simulink model "ROPOD_Control_Control_SIM"  (R2017b)
settings: Solver=VariableStepAuto  StartTime=0.0  StopTime=inf  RelTol=1e-3
values from neighbouring files (symbols this model uses):
  FFtheta_intia = 0    [init_model.m]
  FFxy_mass = 0*80    (= 0)    [init_model.m]
  flock_FFtheta_friction = 50    [init_model.m]
  flock_FFxy_friction = 100    [init_model.m]
  I_fhz_ddelta_cntr = 0    [init_model.m]
  I_fhz_dtheta_cntr = 0.3    [init_model.m]
  I_fhz_dtheta_flock_cntr = 0.1    [init_model.m]
  I_fhz_dvarphi_cntr = 0    [init_model.m]
  I_fhz_dxdy_cntr = 0.25    [init_model.m]
  I_fhz_dxdy_flock_cntr = 0.1    [init_model.m]
  K_gain_ddelta_cntr = 0.1    [init_model.m]
  K_gain_dtheta_cntr = 150    [init_model.m]
  K_gain_dtheta_flock_cntr = 100    [init_model.m]
  K_gain_dvarphi_cntr = 0.05    [init_model.m]
  K_gain_dxdy_cntr = 200    [init_model.m]
  K_gain_dxdy_flock_cntr = 200    [init_model.m]
  LL_wp_fhz_ddelta_cntr = 2    [init_model.m]
  LL_wp_fhz_dtheta_cntr = 20    [init_model.m]
  LL_wp_fhz_dtheta_flock_cntr = 20    [init_model.m]
  LL_wp_fhz_dvarphi_cntr = 10    [init_model.m]
  LL_wp_fhz_dxdy_cntr = 20    [init_model.m]
  LL_wp_fhz_dxdy_flock_cntr = 20    [init_model.m]
  LL_wz_fhz_ddelta_cntr = 2    [init_model.m]
  LL_wz_fhz_dtheta_cntr = 20    [init_model.m]
  LL_wz_fhz_dtheta_flock_cntr = 20    [init_model.m]
  LL_wz_fhz_dvarphi_cntr = 2    [init_model.m]
  LL_wz_fhz_dxdy_cntr = 20    [init_model.m]
  LL_wz_fhz_dxdy_flock_cntr = 20    [init_model.m]
  LPF_fhz_ddelta_cntr = 50    [init_model.m]
  LPF_fhz_ddelta_meas = 50    [init_model.m]
  LPF_fhz_dtheta_cntr = 100    [init_model.m]
  LPF_fhz_dtheta_flock_cntr = 40    [init_model.m]
  LPF_fhz_dvarphi_cntr = 50    [init_model.m]
  LPF_fhz_dvarphi_meas = 50    [init_model.m]
  LPF_fhz_dxdy_cntr = 100    [init_model.m]
  LPF_fhz_dxdy_flock_cntr = 40    [init_model.m]
  max_flock_acc_theta = 0.5    [init_model.m]
  max_flock_acc_xy = 0.5    [init_model.m]
  max_flock_vel_theta = 1.0    (= 1)    [init_model.m]
  max_flock_vel_xy = 1.0    (= 1)    [init_model.m]
  max_hw_tau = 7.0    (= 7)    [init_model.m]
  max_ropod_acc_theta = 1.6    [init_model.m]
  max_ropod_acc_xy = 2.0    (= 2)    [init_model.m]
  max_ropod_sw_force = 500    [init_model.m]
  max_ropod_sw_tau = 250    [init_model.m]
  max_ropod_vel_theta = 1.6    [init_model.m]
  max_ropod_vel_xy = 2.0    (= 2)    [init_model.m]
  max_sw_current = 10    [init_model.m]
  Nagents = 2    [init_model.m]
  Nwheels = 4    [Jqwl_numeric_function.m]    (also in S_matrix.m; extract_kinmodel_parameters.m; init_model.m; tau_optimal_dist_vec_fun.m)
  pivot_offs_sws = [0.0243    0.4689    0.3384    5.9050]    [init_model.m]
  ropod_kinmodel_pv = struct2array(ropod_kinmodel_param)    [set_ropod_KinModparams.m]
  ropod_position_inflock = [-1 0 3.1416]    [init_model.m]
  SW_COM1_ENABLE1 = hex2dec('0001')    [init_model.m]
  SW_COM1_ENABLE2 = hex2dec('0002')    [init_model.m]
  SW_COM1_MODE_TORQUE = bitshift(hex2dec('0000'),2)    [init_model.m]
  SW_COM1_MODE_VELOCITY = bitshift(hex2dec('0002'),2)    [init_model.m]
  SW_COM1_USE_TS = hex2dec('8000')    [init_model.m]
  Tinit = 2    [init_model.m]
  Ts = 0.001    [init_model.m]
  Tsflck = 0.01    [init_model.m]
undefined symbols (not defined in the file or in its folder): DiscIntNeverNeededParam, sw_tau_2_curr
libraries: simulink x80, cstblocks x30, dspsigops x12, dspnetwork x4
(part 1 of 6)
settings Model: Creator=cesar  LastModifiedBy=cesar
settings OptimizationCC: DefaultParameterBehavior=Inlined  UseFloatMulNetSlope=on  InlineInvariantSignals=on  EfficientFloat2IntCast=on
settings DebuggingCC: UnderSpecifiedDataTypeMsg=warning
settings HardwareCC: ProdBitPerLong=64  ProdHWDeviceType=Intel->x86-64 (Linux 64)
settings RTWCC: GenCodeOnly=on  BuildConfiguration=Faster Runs
settings GRTTargetCC: MatFileLogging=off  SupportNonFinite=off

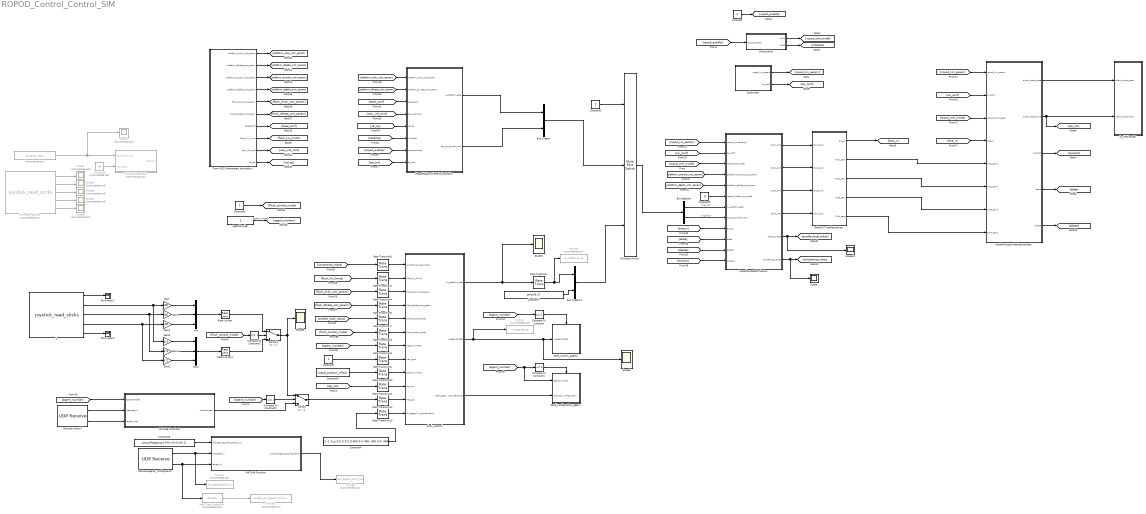
== system ROPOD_Control_Control_SIM ==
  " " : S-Function  Commented=on  FunctionName=joystick_read  SFunctionDeploymentMode=off  EnableBusSupport=off  mask(Legacy Function){SFunctionSpec=double y1 = read_joystick(), ShowSpec=off}
      mask prompts: ShowSpec "Display function specification"
      mask help:
      | This block allows you to call the legacy functions specified by the following Legacy Code Tool definition:
      | def.SFunctionName = 'joystick_read';
      | def.OutputFcnSpec = 'double y1 = read_joystick()';
      | def.StartFcnSpec = 'void init()';
      | def.HeaderFiles = {'joystick.h', 'stdio.h', 'ncurses.h', 'gamepad.h'};
      | def.SourceFiles = {'joystick.c'};
      | def.HostLibFiles = {'libgamepad.so.1'};
      mask Help: <p>This block was generated automatically by the Legacy Code Tool. For detailed help on this tool, call<a href="matlab:legacy_code('help')"> legacy_code('help')</a>.</p>
      mask Callback ShowSpec:
      | if strcmp(get_param(gcbh, 'ShowSpec'), 'on')
      |   set_param(gcbh, 'MaskDisplay', sprintf('fprintf(''%s'');', get_param(gcbh, 'SFunctionSpec')));
      | else
      |   set_param(gcbh, 'MaskDisplay', sprintf('fprintf(''%s'');', get_param(gcbh, 'FunctionName')));
      | end
      mask Display: fprintf('joystick_read');
  " 1" : S-Function  FunctionName=joystick_read_sticks  SFunctionDeploymentMode=off  EnableBusSupport=off  mask(Legacy Function){SFunctionSpec=double y1 = read_joystick(), ShowSpec=off}
      mask prompts: ShowSpec "Display function specification"
      mask help:
      | This block allows you to call the legacy functions specified by the following Legacy Code Tool definition:
      | def.SFunctionName = 'joystick_read';
      | def.OutputFcnSpec = 'double y1 = read_joystick()';
      | def.StartFcnSpec = 'void init()';
      | def.HeaderFiles = {'joystick.h', 'stdio.h', 'ncurses.h', 'gamepad.h'};
      | def.SourceFiles = {'joystick.c'};
      | def.HostLibFiles = {'libgamepad.so.1'};
      mask Help: <p>This block was generated automatically by the Legacy Code Tool. For detailed help on this tool, call<a href="matlab:legacy_code('help')"> legacy_code('help')</a>.</p>
      mask Callback ShowSpec:
      | if strcmp(get_param(gcbh, 'ShowSpec'), 'on')
      |   set_param(gcbh, 'MaskDisplay', sprintf('fprintf(''%s'');', get_param(gcbh, 'SFunctionSpec')));
      | else
      |   set_param(gcbh, 'MaskDisplay', sprintf('fprintf(''%s'');', get_param(gcbh, 'FunctionName')));
      | end
      mask Display: fprintf('joystick_read_sticks');
  AgentNumber : Constant
  Bus Creator : BusCreator  Inputs=2
  Bus Creator1 : BusCreator  Inputs=2
  Bus Selector : BusSelector  OutputSignals=signal1,signal2
  Compare To Constant : simulink/Logic and Bit Operations/Compare To Constant  relop===  const=1  OutDataTypeStr=boolean
  Compare To Constant1 : simulink/Logic and Bit Operations/Compare To Constant  relop=~=  const=1  OutDataTypeStr=boolean
  Compare To Constant2 : simulink/Logic and Bit Operations/Compare To Constant  relop===  const=1  OutDataTypeStr=boolean
  Compare To Constant3 : simulink/Logic and Bit Operations/Compare To Constant  relop===  const=1  OutDataTypeStr=boolean
  Constant : Constant
  Constant1 : Constant
  Constant2 : Constant  Value=2
  Constant3 : Constant  Value=3
  Constant4 : Constant  Value=[1 -1 0 pi 0.0 0.0 0.0 400 0 0 400 -400 0 0 -400]
  Constant5 : Constant
  Constant6 : Constant  Commented=on  Value=30
  Constant7 : Constant  Value=zeros(3,1)
  Constant8 : Constant  Value=zeros((Nagents-1)*(1+3+3+8),1)
  Constant9 : Constant  Value=ropod_position_inflock
  Data Type Conversion : DataTypeConversion  Commented=on  OutDataTypeStr=double
  EtherCAT Interface empty : Subsystem
  Flock_Control : Subsystem
  From ROS (Parameters and topics) : Subsystem
  Gain : Gain  Gain=200
  Gain1 : Gain  Gain=200
  Gain2 : Gain  Gain=100
  Gain3 : Gain  Gain=0.2
  Gain4 : Gain  Gain=0.5
  Gain5 : Gain  Gain=0.5
  Initialization : Subsystem
  MATLAB Function : MATLAB Function  TreatAsAtomicUnit=on
  MATLAB Function1 : MATLAB Function  TreatAsAtomicUnit=on
  MATLAB Function2 : MATLAB Function  Commented=on  TreatAsAtomicUnit=on
  Multiport Switch : MultiPortSwitch  Inputs=2
  Mux : Mux  Inputs=3
  Mux1 : Mux  Inputs=3
  Rate Limiter : RateLimiter  RisingSlewLimit=200  FallingSlewLimit=-200  SampleTimeMode=inherited
  Rate Limiter1 : RateLimiter  SampleTimeMode=inherited
  Rate Transition : RateTransition  OutPortSampleTime=Ts
  Rate Transition{1..5,7..13} (12 alike) : RateTransition  OutPortSampleTime=Tsflck
  Recieve agents_configuration : dspnetwork/UDP Receive  localURL='0.0.0.0'  localPort=25002  remoteURL='0.0.0.0'  remotePort=-1  recvBufferSize=8192  dims=(1+1+3+8)  signalDatatype=double  isVarSize=off  showBlockingTime=on  blockingTime=0  sampletime=Ts  blockPlatform=HOST
      settings: SourceProductName=DSP System Toolbox  SourceProductBaseCode=DS
  Recieve wrench : dspnetwork/UDP Receive  localURL='0.0.0.0'  localPort=25001  remoteURL='0.0.0.0'  remotePort=-1  recvBufferSize=8192  dims=3*(Nagents-1)  signalDatatype=double  isVarSize=off  showBlockingTime=on  blockingTime=0  sampletime=Ts  blockPlatform=HOST
      settings: SourceProductName=DSP System Toolbox  SourceProductBaseCode=DS
  RopodPlatformVelocityController : Subsystem
  RopodProcessWheelSensorData : Subsystem
  RopodTorqueDistribution : Subsystem
  S-Function Builder : S-Function  Commented=on  FunctionName=joystick_read_sticks  SFunctionModules=joystick_read_sticks_wrapper joystick gamepad  SFunctionDeploymentMode=off  EnableBusSupport=off  mask(S-Function Builder){}
      mask help: Simulink:masks:SFunctionBuilder_MD
      mask init:
      | val = [[.9  0.75 0.75 1 1 .9 .9 1]',[1 1 0.75 0.75 .9 .9 1 .9]'];try , sys = get_param(gcb,'SfunBuilderFcnName');if isempty(sys), sys = get_param(gcb,'FunctionName'); end,catch, sys = get_param(gcb,'FunctionName'); end
      settings: CopyFcn=set_param(gcbh,'LinkStatus','none')  PreSaveFcn=try, set_param(gcb,'FunctionName','joystick_read_sticks'), end  OpenFcn=sfunctionwizard(gcbh)
      mask Display: plot(val(:,1),val(:,2)),disp(sys), port_label('output',1,'button'), port_label('output',2,'outX1'), port_label('output',3,'outY1'), port_label('output',4,'outX2'), port_label('output',5,'outY2')
  Scope{,2..3,9..10} (5 alike) : Scope
  Scope{1,4..8} (6 alike) : Scope  Commented=on
  Send_configuration_agent : Subsystem
  Send_wrench_agents : Subsystem
  Subsystem : Subsystem
  Switch : Switch  Criteria=u2 > Threshold
  Switch1 : Switch  Criteria=u2 > Threshold
  Terminator2 : Terminator
  Terminator3 : Terminator
  To File2 : ToFile  Commented=on  Filename=w_platform_sp  MatrixName=w_platform_sp
  To File4 : ToFile  Commented=on  Filename=ext_agent_conf_in  MatrixName=ext_agent_conf_in
  To File5 : ToFile  Commented=on  Filename=length_ext_agent_conf_in  MatrixName=length_ext_agent_conf_in
  To File6 : ToFile  Commented=on  Filename=ext_agent_conf_out  MatrixName=ext_agent_conf_out
  To File7 : ToFile  Commented=on  Filename=w_agents_sp  MatrixName=w_agents_sp
  to_ROS empty : Subsystem
  wires:
  [sw_conf] -> RopodProcessWheelSensorData/2(sw_conf)
  RopodProcessWheelSensorData/2(odom_robot_twist) -> to_ROS empty/2(odom_robot_twist), [dqr_loc]
  Constant5/1 -> [flock_control_mode]
  RopodTorqueDistribution/3(SW3_cmd) -> EtherCAT Interface empty/3(SW3_cmd)
  RopodProcessWheelSensorData/1(odom_robot_pose) -> to_ROS empty/1(odom_robot_pose)
  Constant/1 -> [ropod_enable]
  RopodTorqueDistribution/1(SW1_cmd) -> EtherCAT Interface empty/1(SW1_cmd)
  [ropod_cntr_mode] -> RopodProcessWheelSensorData/3(ropod_cntr_mode)
  Initialization/1(Out1) -> [ropod_cntr_mode]
  Subsystem/2(sw_conf) -> [sw_conf]
  RopodTorqueDistribution/2(SW2_cmd) -> EtherCAT Interface empty/2(SW2_cmd)
  [ropod_enable] -> Initialization/1(ropod_enable)
  [ena_w] -> RopodProcessWheelSensorData/4(ena_w)
  RopodProcessWheelSensorData/3(dvarphi) -> [dvarphi]
  Constant2/1 -> Multiport Switch/1
  Subsystem/1(ropod_kin_param) -> [ropod_kin_param]
  AgentNumber/1 -> [agent_number]  "agent_number"
  RopodProcessWheelSensorData/5(ddelta) -> [ddelta]
  RopodTorqueDistribution/4(SW4_cmd) -> EtherCAT Interface empty/4(SW4_cmd)
  RopodProcessWheelSensorData/4(delta) -> [delta]
  [ropod_kin_param] -> RopodProcessWheelSensorData/1(ropod_kin_param)
  Initialization/2(Out2) -> [initialize]
  EtherCAT Interface empty/1(ena_w) -> [ena_w]
  EtherCAT Interface empty/2(SW1_sens) -> RopodProcessWheelSensorData/5(SW1_sens)
  EtherCAT Interface empty/3(SW2_sens) -> RopodProcessWheelSensorData/6(SW2_sens)
  EtherCAT Interface empty/4(SW3_sens) -> RopodProcessWheelSensorData/7(SW3_sens)
  EtherCAT Interface empty/5(SW4_sens) -> RopodProcessWheelSensorData/8(SW4_sens)
  " "/1 -> MATLAB Function2/1(gamepad_input), Scope1/1
  S-Function Builder/1 -> Scope4/1
  S-Function Builder/2 -> Scope5/1
  S-Function Builder/3 -> Scope6/1
  S-Function Builder/4 -> Scope7/1
  S-Function Builder/5 -> Scope8/1
  Constant6/1 -> MATLAB Function2/2(max_force)
  [delta] -> RopodTorqueDistribution/10(delta)
  Bus Selector/1 -> RopodTorqueDistribution/7(w_platform_setp)  "<signal1>"
  [ropod_cntr_mode] -> RopodTorqueDistribution/3(ropod_cntr_mode)
  [ropod_kin_param] -> RopodTorqueDistribution/1(ropod_kinmodel_pv)
  Multiport Switch/1 -> Bus Selector/1
  [ddelta] -> RopodTorqueDistribution/11(ddelta)
  Bus Selector/2 -> RopodTorqueDistribution/8(dqr_sp_dvarphi_cntr)  "<signal2>"
  [ena_w] -> RopodTorqueDistribution/9(ena_w)
  Constant3/1 -> RopodTorqueDistribution/6(ropod_wheel_cntr_mode)
  RopodTorqueDistribution/5(enable_robot) -> Scope10/1, [enable_local_robot]
  [platform_dvarphi_cntr_param] -> RopodTorqueDistribution/4(platform_dvarphi_cntr_param)
  [sw_conf] -> RopodTorqueDistribution/2(sw_conf)
  [dvarphi] -> RopodTorqueDistribution/12(dvarphi)
  [platform_ddelta_cntr_param] -> RopodTorqueDistribution/5(platform_ddelta_cntr_param)
  RopodTorqueDistribution/6(constraints_robot) -> Scope/1, [constraints_robot]
  From ROS (Parameters and topics)/1(platform_dxdy_cntr_param) -> [platform_dxdy_cntr_param]
  From ROS (Parameters and topics)/9(new_vel_cmd) -> [new_vel_cmd]
  From ROS (Parameters and topics)/4(platform_ddelta_cntr_param) -> [platform_ddelta_cntr_param]
  From ROS (Parameters and topics)/2(platform_dtheta_cntr_param) -> [platform_dtheta_cntr_param]
  From ROS (Parameters and topics)/7(base_conf) -> [base_conf]
  From ROS (Parameters and topics)/8(flock_kin_limits) -> [flock_kin_limits]
  From ROS (Parameters and topics)/6(flock_dtheta_cntr_param) -> [flock_dtheta_cntr_param]
  From ROS (Parameters and topics)/5(flock_dxdy_cntr_param) -> [flock_dxdy_cntr_param]
  From ROS (Parameters and topics)/3(platform_dvarphi_cntr_param) -> [platform_dvarphi_cntr_param]
  From ROS (Parameters and topics)/10(vel_sp) -> [vel_sp]
  [base_conf] -> RopodPlatformVelocityController/3(base_conf)
  [platform_dtheta_cntr_param] -> RopodPlatformVelocityController/2(platform_dtheta_cntr_param)
  [new_vel_cmd] -> RopodPlatformVelocityController/4(new_vel_cmd)
  [vel_sp] -> RopodPlatformVelocityController/5(vel_sp)
  [initialize] -> RopodPlatformVelocityController/6(initialize)
  RopodPlatformVelocityController/2(dqr_sp_dvarphi_cntr) -> Bus Creator/2
  Bus Creator/1 -> Multiport Switch/2
  [dqr_loc] -> RopodPlatformVelocityController/8(dqr_loc)
  [platform_dxdy_cntr_param] -> RopodPlatformVelocityController/1(platform_dxdy_cntr_param)
  [ropod_enable] -> RopodPlatformVelocityController/7(ropod_enable)
  RopodPlatformVelocityController/1(w_platform_setp) -> Bus Creator/1
  Rate Transition12/1 -> Flock_Control/11(flock_sp)
  [dqr_loc] -> Rate Transition11/1
  Bus Creator1/1 -> Multiport Switch/3
  Gain1/1 -> Mux/2
  [agent_number] -> Rate Transition9/1
  Constant7/1 -> Bus Creator1/2
  Gain2/1 -> Mux/3
  Rate Transition5/1 -> Flock_Control/4(flock_dtheta_cntr_param)
  Recieve wrench/2 -> MATLAB Function1/3(length_msg)
  Rate Transition2/1 -> Flock_Control/8(new_cmd)
  [constraints_robot] -> Rate Transition3/1
  Rate Transition4/1 -> Flock_Control/3(flock_dxdy_cntr_param)
  [agent_number] -> Compare To Constant/1
  Flock_Control/2(w_agents_setp) -> To File7/1, Scope3/1, Send_wrench_agents/1(w_agents_setp)
  [flock_dtheta_cntr_param] -> Rate Transition5/1
  Rate Transition7/1 -> Flock_Control/5(enable_local_robot)
  " 1"/2 -> Gain5/1, Gain/1
  Compare To Constant1/1 -> Send_configuration_agent/Enable
  [flock_dxdy_cntr_param] -> Rate Transition4/1
  [agent_number] -> Compare To Constant2/1
  Rate Transition8/1 -> Flock_Control/6(flock_control_mode)
  Data Type Conversion/1 -> To File5/1
  " 1"/1 -> Terminator2/1
  [agent_number] -> MATLAB Function1/1(AgentNumber)
  Gain/1 -> Mux/1
  Mux/1 -> Rate Limiter/1
  Switch/1 -> Rate Transition12/1
  Rate Transition3/1 -> Flock_Control/1(constraints_local_robot)
  [flock_kin_limits] -> Rate Transition1/1
  Compare To Constant2/1 -> Switch/2
  Constant1/1 -> Rate Transition2/1
  " 1"/3 -> Gain4/1, Gain1/1
  [flock_control_mode] -> Rate Transition8/1
  Flock_Control/3(local_agent_configuration) -> Send_configuration_agent/2(local_agent_configuration)
  Rate Transition11/1 -> Flock_Control/10(dqr_loc)
  " 1"/4 -> Gain3/1, Gain2/1
  [enable_local_robot] -> Rate Transition7/1
  Rate Transition1/1 -> Flock_Control/2(flock_kin_limits)
  MATLAB Function/1(out_ext_agents_configuration) -> To File6/1
  Compare To Constant/1 -> Send_wrench_agents/Enable
  Rate Transition9/1 -> Flock_Control/7(agent_number)
  Constant9/1 -> Rate Transition10/1
  Flock_Control/1(w_platform_setp) -> Scope2/1, Rate Transition/1
  Constant8/1 -> MATLAB Function/1(ext_agents_configuration_ini)
  Recieve wrench/1 -> MATLAB Function1/2(message_in)
  Rate Transition10/1 -> Flock_Control/9(position_inflock)
  MATLAB Function1/1(WrenchAgent) -> Switch/3
  Rate Transition13/1 -> Flock_Control/12(ext_agents_configuration)
  [agent_number] -> Send_configuration_agent/1(agent_number), Compare To Constant1/1
  Rate Transition/1 -> To File2/1, Bus Creator1/1
  " 1"/5 -> Terminator3/1
  Recieve agents_configuration/1 -> To File4/1, MATLAB Function/2(message_in)
  Recieve agents_configuration/2 -> Data Type Conversion/1, MATLAB Function/3(length_in)
  Constant4/1 -> Rate Transition13/1
  [flock_control_mode] -> Compare To Constant3/1
  Compare To Constant3/1 -> Switch1/2
  Rate Limiter/1 -> Switch1/1
  Switch1/1 -> Switch/1, Scope9/1
  Gain5/1 -> Mux1/1
  Gain4/1 -> Mux1/2
  Gain3/1 -> Mux1/3
  Mux1/1 -> Rate Limiter1/1
  Rate Limiter1/1 -> Switch1/3

== system ROPOD_Control_Control_SIM/EtherCAT Interface empty ==
  SW1_cmd : Inport
  SW2_cmd : Inport  Port=2
  SW3_cmd : Inport  Port=3
  SW4_cmd : Inport  Port=4
  Constant : Constant  Value=[1 1 1 1]
  empywheel : Subsystem
  empywheel1 : Subsystem
  empywheel2 : Subsystem
  empywheel3 : Subsystem
  ena_w : Outport
  SW1_sens : Outport  Port=2
  SW2_sens : Outport  Port=3
  SW3_sens : Outport  Port=4
  SW4_sens : Outport  Port=5
  wires:
  empywheel1/1(SW4_sens) -> SW2_sens/1  "SW2_sens"
  empywheel2/1(SW4_sens) -> SW3_sens/1  "SW3_sens"
  SW4_cmd/1 -> empywheel3/1(SW4_cmd)
  SW2_cmd/1 -> empywheel1/1(SW4_cmd)
  SW3_cmd/1 -> empywheel2/1(SW4_cmd)
  SW1_cmd/1 -> empywheel/1(SW4_cmd)
  empywheel/1(SW4_sens) -> SW1_sens/1  "SW1_sens"
  empywheel3/1(SW4_sens) -> SW4_sens/1  "SW4_sens"
  Constant/1 -> ena_w/1

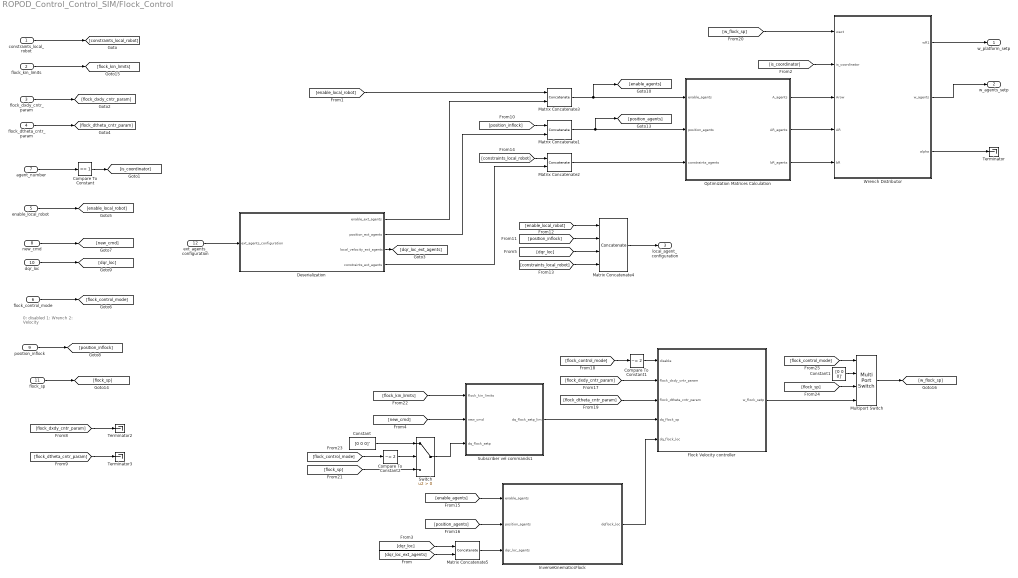
== system ROPOD_Control_Control_SIM/Flock_Control ==
  note: 0: disabled
      | 1: Wrench
      | 2: Velocity
  constraints_local_robot : Inport
  flock_kin_limits : Inport  Port=2
  flock_dxdy_cntr_param : Inport  Port=3
  flock_dtheta_cntr_param : Inport  Port=4
  enable_local_robot : Inport  Port=5
  flock_control_mode : Inport  Port=6
  agent_number : Inport  Port=7
  new_cmd : Inport  Port=8
  position_inflock : Inport  Port=9
  dqr_loc : Inport  Port=10
  flock_sp : Inport  Port=11
  ext_agents_configuration : Inport  Port=12
  Compare To Constant : simulink/Logic and Bit Operations/Compare To Constant  relop===  const=1  OutDataTypeStr=boolean
  Compare To Constant1 : simulink/Logic and Bit Operations/Compare To Constant  relop=~=  const=2  OutDataTypeStr=boolean
  Compare To Constant2 : simulink/Logic and Bit Operations/Compare To Constant  relop=~=  const=2  OutDataTypeStr=boolean
  Constant : Constant  Value=[0 0 0]'
  Constant1 : Constant  Value=[0 0 0]'
  Deserialization : MATLAB Function  TreatAsAtomicUnit=on
  Flock Velocity controller : Subsystem
  InverseKinematicsFlock : MATLAB Function  TreatAsAtomicUnit=on
  Matrix Concatenate1 : Concatenate  Mode=Multidimensional array  ConcatenateDimension=2
  Matrix Concatenate2 : Concatenate  Mode=Multidimensional array  ConcatenateDimension=2
  Matrix Concatenate3 : Concatenate  Mode=Multidimensional array  ConcatenateDimension=2
  Matrix Concatenate4 : Concatenate  NumInputs=4  Mode=Multidimensional array
  Matrix Concatenate5 : Concatenate  Mode=Multidimensional array
  Multiport Switch : MultiPortSwitch  DataPortOrder=Zero-based contiguous
  Optimization Matrices Calculation : MATLAB Function  TreatAsAtomicUnit=on
  Subscriber vel commands1 : Subsystem
  Switch : Switch  Criteria=u2 > Threshold
  Terminator : Terminator
  Terminator2 : Terminator
  Terminator3 : Terminator
  Wrench Distributor : MATLAB Function  TreatAsAtomicUnit=on
  w_platform_setp : Outport
  w_agents_setp : Outport  Port=2
  local_agent_configuration : Outport  Port=3
  wires:
  constraints_local_robot/1 -> [constraints_local_robot]
  Wrench Distributor/1(wR1) -> w_platform_setp/1
  agent_number/1 -> Compare To Constant/1
  [is_coordinator] -> Wrench Distributor/2(is_coordinator)
  Wrench Distributor/2(w_agents) -> w_agents_setp/1
  Wrench Distributor/3(alpha) -> Terminator/1
  flock_dxdy_cntr_param/1 -> [flock_dxdy_cntr_param]
  flock_dtheta_cntr_param/1 -> [flock_dtheta_cntr_param]
  ext_agents_configuration/1 -> Deserialization/1(ext_agents_configuration)
  Optimization Matrices Calculation/1(A_agents) -> Wrench Distributor/3(Arow)
  Optimization Matrices Calculation/2(AR_agents) -> Wrench Distributor/4(AR)
  Optimization Matrices Calculation/3(bR_agents) -> Wrench Distributor/5(bR)
  Deserialization/1(enable_ext_agents) -> Matrix Concatenate3/2
  Deserialization/4(constraints_ext_agents) -> Matrix Concatenate2/2
  Deserialization/2(position_ext_agents) -> Matrix Concatenate1/2
  Matrix Concatenate2/1 -> Optimization Matrices Calculation/3(constraints_agents)
  Matrix Concatenate1/1 -> [position_agents], Optimization Matrices Calculation/2(position_agents)
  Matrix Concatenate3/1 -> [enable_agents], Optimization Matrices Calculation/1(enable_agents)
  dqr_loc/1 -> [dqr_loc]
  enable_local_robot/1 -> [enable_local_robot]
  [enable_local_robot] -> Matrix Concatenate3/1
  flock_control_mode/1 -> [flock_control_mode]
  [flock_dxdy_cntr_param] -> Terminator2/1
  [flock_dtheta_cntr_param] -> Terminator3/1
  Matrix Concatenate4/1 -> local_agent_configuration/1
  position_inflock/1 -> [position_inflock]
  [position_inflock] -> Matrix Concatenate1/1
  [position_inflock] -> Matrix Concatenate4/2
  Compare To Constant/1 -> [is_coordinator]
  Deserialization/3(local_velocity_ext_agents) -> [dqr_loc_ext_agents]
  [dqr_loc_ext_agents] -> Matrix Concatenate5/2
  [dqr_loc] -> Matrix Concatenate5/1
  Matrix Concatenate5/1 -> InverseKinematicsFlock/3(dqr_loc_agents)
  [dqr_loc] -> Matrix Concatenate4/3
  [enable_local_robot] -> Matrix Concatenate4/1
  [constraints_local_robot] -> Matrix Concatenate4/4
  [constraints_local_robot] -> Matrix Concatenate2/1
  [position_agents] -> InverseKinematicsFlock/2(position_agents)
  [enable_agents] -> InverseKinematicsFlock/1(enable_agents)
  InverseKinematicsFlock/1(dqflock_loc) -> Flock Velocity controller/5(dq_flock_loc)
  [flock_dxdy_cntr_param] -> Flock Velocity controller/2(flock_dxdy_cntr_param)
  [flock_dtheta_cntr_param] -> Flock Velocity controller/3(flock_dtheta_cntr_param)
  [flock_control_mode] -> Compare To Constant1/1
  Compare To Constant1/1 -> Flock Velocity controller/1(disable)
  [w_flock_sp] -> Wrench Distributor/1(wact)
  flock_sp/1 -> [flock_sp]
  flock_kin_limits/1 -> [flock_kin_limits]
  [flock_kin_limits] -> Subscriber vel commands1/1(flock_kin_limits)
  Subscriber vel commands1/1(dq_flock_setp_lim) -> Flock Velocity controller/4(dq_flock_sp)
  Compare To Constant2/1 -> Switch/2
  [flock_sp] -> Switch/3
  [flock_control_mode] -> Compare To Constant2/1
  Constant/1 -> Switch/1
  [flock_sp] -> Multiport Switch/3
  [flock_control_mode] -> Multiport Switch/1
  Constant1/1 -> Multiport Switch/2
  Flock Velocity controller/1(w_flock_setp) -> Multiport Switch/4
  Multiport Switch/1 -> [w_flock_sp]
  Switch/1 -> Subscriber vel commands1/3(dq_flock_setp)
  new_cmd/1 -> [new_cmd]
  [new_cmd] -> Subscriber vel commands1/2(new_cmd)

== system ROPOD_Control_Control_SIM/From ROS (Parameters and topics) ==
  note: doing the transformation with the angle from odometry data helps
      | to keep the robot better align during the Identification, especially because
      | we do not have any absolute reference
  Constant1 : Constant
  Controllers conf : Subsystem
  From Workspace1 : FromWorkspace  VariableName=qrefdot  SampleTime=Ts
  Gain1 : Gain
  ROS base conf : Subsystem
  Selector1 : Selector  InputPortWidth=3  IndexOptions=Index vector (dialog)  Indices=3  OutputSizes=1
  flock kin limits : Subsystem
  rot_matrix2 : MATLAB Function  TreatAsAtomicUnit=on
  platform_dxdy_cntr_param : Outport
  platform_dtheta_cntr_param : Outport  Port=2
  platform_dvarphi_cntr_param : Outport  Port=3
  platform_ddelta_cntr_param : Outport  Port=4
  flock_dxdy_cntr_param : Outport  Port=5
  flock_dtheta_cntr_param : Outport  Port=6
  base_conf : Outport  Port=7
  flock_kin_limits : Outport  Port=8
  new_vel_cmd : Outport  Port=9
  vel_sp : Outport  Port=10
  wires:
  Controllers conf/1(platform_dxdy_cntr_param) -> platform_dxdy_cntr_param/1
  Constant1/1 -> new_vel_cmd/1
  Gain1/1 -> vel_sp/1
  ROS base conf/1(base_conf) -> base_conf/1
  From Workspace1/1 -> Selector1/1, rot_matrix2/1(dqr_glb)
  Controllers conf/3(platform_dvarphi_cntr_param) -> platform_dvarphi_cntr_param/1
  Controllers conf/2(platform_dtheta_cntr_param) -> platform_dtheta_cntr_param/1
  Selector1/1 -> rot_matrix2/2(theta)
  rot_matrix2/1(dqr_loc) -> Gain1/1
  Controllers conf/4(platform_ddelta_cntr_param) -> platform_ddelta_cntr_param/1
  Controllers conf/5(flock_dxdy_cntr_param) -> flock_dxdy_cntr_param/1
  Controllers conf/6(flock_dtheta_cntr_param) -> flock_dtheta_cntr_param/1
  flock kin limits/1(flock_kin_limits) -> flock_kin_limits/1

== system ROPOD_Control_Control_SIM/Initialization ==
  ropod_enable : Inport
  Allow Tinit seconds for initialization : simulink/Logic and Bit Operations/Compare To Constant  relop=<  const=Tinit  OutDataTypeStr=boolean
  Constant : Constant  Value=2
  Constant1 : Constant
  Constant2 : Constant  Value=0
  Digital Clock : DigitalClock  SampleTime=Ts
  Gain : Gain
  Gain1 : Gain  OutDataTypeStr=double
  Switch : Switch  Criteria=u2 > Threshold
  Switch1 : Switch  Criteria=u2 > Threshold
  Out1 : Outport
  Out2 : Outport  Port=2
  wires:
  Switch/1 -> Switch1/1
  Constant1/1 -> Switch/3
  Switch1/1 -> Gain/1
  Digital Clock/1 -> Allow Tinit seconds for initialization/1
  Allow Tinit seconds for initialization/1 -> Gain1/1, Switch/2
  Constant2/1 -> Switch1/3
  Constant/1 -> Switch/1
  ropod_enable/1 -> Switch1/2
  Gain/1 -> Out1/1
  Gain1/1 -> Out2/1

== system ROPOD_Control_Control_SIM/RopodPlatformVelocityController ==
  platform_dxdy_cntr_param : Inport
  platform_dtheta_cntr_param : Inport  Port=2
  base_conf : Inport  Port=3
  new_vel_cmd : Inport  Port=4
  vel_sp : Inport  Port=5
  initialize : Inport  Port=6
  ropod_enable : Inport  Port=7
  dqr_loc : Inport  Port=8
  Logical Operator : Logic  Operator=OR  AllPortsSameDT=off  OutDataTypeStr=boolean
  Logical Operator1 : Logic  Operator=NOT  AllPortsSameDT=off  OutDataTypeStr=boolean
  Platorm Velocity controller : Subsystem
  Subscriber vel commands1 : Subsystem
  w_platform_setp : Outport
  dqr_sp_dvarphi_cntr : Outport  Port=2
  wires:
  platform_dxdy_cntr_param/1 -> [platform_dxdy_cntr_param]
  platform_dtheta_cntr_param/1 -> [platform_dtheta_cntr_param]
  vel_sp/1 -> Subscriber vel commands1/3(dq_setp)
  base_conf/1 -> Subscriber vel commands1/1(base_conf)
  new_vel_cmd/1 -> Subscriber vel commands1/2(new_cmd)
  [platform_dxdy_cntr_param] -> Platorm Velocity controller/2(platform_dxdy_cntr_param)
  dqr_loc/1 -> Platorm Velocity controller/5(dqr_loc)
  Subscriber vel commands1/1(dq_loc_sp) -> dqr_sp_dvarphi_cntr/1, Platorm Velocity controller/4(dqr_sp)
  Platorm Velocity controller/1(w_platform_setp) -> w_platform_setp/1
  ropod_enable/1 -> Logical Operator1/1
  Logical Operator1/1 -> Logical Operator/2
  Logical Operator/1 -> Platorm Velocity controller/1(reset_int)
  initialize/1 -> Logical Operator/1
  [platform_dtheta_cntr_param] -> Platorm Velocity controller/3(platform_dtheta_cntr_param)

== system ROPOD_Control_Control_SIM/RopodProcessWheelSensorData ==
  ropod_kin_param : Inport
  sw_conf : Inport  Port=2
  ropod_cntr_mode : Inport  Port=3
  ena_w : Inport  Port=4
  SW1_sens : Inport  Port=5
  SW2_sens : Inport  Port=6
  SW3_sens : Inport  Port=7
  SW4_sens : Inport  Port=8
  Compare To Constant : simulink/Logic and Bit Operations/Compare To Constant  relop=~=  const=1  OutDataTypeStr=boolean
  Odometry and Measurement model 4SW : Subsystem
  ROPOD_4Wheel_sens : Subsystem
  odom_robot_pose : Outport
  odom_robot_twist : Outport  Port=2
  dvarphi : Outport  Port=3
  delta : Outport  Port=4
  ddelta : Outport  Port=5
  wires:
  ropod_kin_param/1 -> Odometry and Measurement model 4SW/1(param_in)
  Odometry and Measurement model 4SW/2(odom_robot_twist) -> odom_robot_twist/1
  SW2_sens/1 -> ROPOD_4Wheel_sens/4(SW2_sens)
  ROPOD_4Wheel_sens/3(ddelta) -> ddelta/1
  Odometry and Measurement model 4SW/1(odom_robot_pose) -> odom_robot_pose/1
  ROPOD_4Wheel_sens/2(delta) -> Odometry and Measurement model 4SW/4(delta), delta/1
  SW4_sens/1 -> ROPOD_4Wheel_sens/6(SW4_sens)
  ROPOD_4Wheel_sens/1(dvarphi) -> Odometry and Measurement model 4SW/3(dvarphi), dvarphi/1
  SW3_sens/1 -> ROPOD_4Wheel_sens/5(SW3_sens)
  SW1_sens/1 -> ROPOD_4Wheel_sens/3(SW1_sens)
  Compare To Constant/1 -> ROPOD_4Wheel_sens/1(disable)
  sw_conf/1 -> ROPOD_4Wheel_sens/2(sw_conf)
  ropod_cntr_mode/1 -> Compare To Constant/1
  ena_w/1 -> Odometry and Measurement model 4SW/2(ena_w)

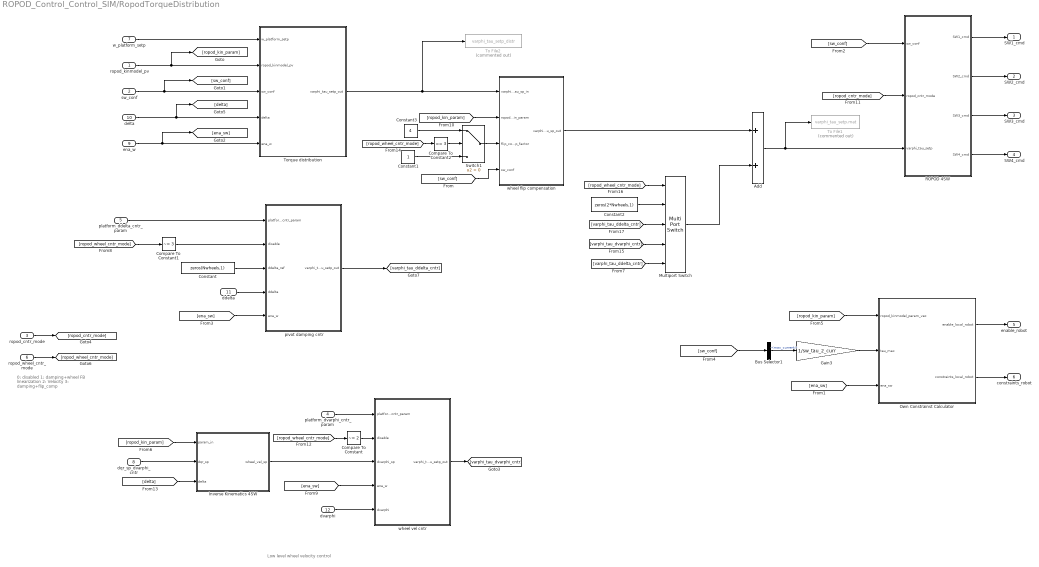
== system ROPOD_Control_Control_SIM/RopodTorqueDistribution ==
  note: Low level wheel velocity control
  note: 0: disabled
      | 1: damping+wheel FB linearization
      | 2: Velocity
      | 3: damping+flip_comp
  ropod_kinmodel_pv : Inport
  sw_conf : Inport  Port=2
  ropod_cntr_mode : Inport  Port=3
  platform_dvarphi_cntr_param : Inport  Port=4
  platform_ddelta_cntr_param : Inport  Port=5
  ropod_wheel_cntr_mode : Inport  Port=6
  w_platform_setp : Inport  Port=7
  dqr_sp_dvarphi_cntr : Inport  Port=8
  ena_w : Inport  Port=9
  delta : Inport  Port=10
  ddelta : Inport  Port=11
  dvarphi : Inport  Port=12
  Add : Sum
  Bus Selector1 : BusSelector  OutputSignals=max_current
  Compare To Constant : simulink/Logic and Bit Operations/Compare To Constant  relop=~=  const=2  OutDataTypeStr=boolean
  Compare To Constant1 : simulink/Logic and Bit Operations/Compare To Constant  relop=~=  const=3  OutDataTypeStr=boolean
  Compare To Constant2 : simulink/Logic and Bit Operations/Compare To Constant  relop===  const=3  OutDataTypeStr=boolean
  Constant : Constant  Value=zeros(Nwheels,1)
  Constant1 : Constant
  Constant2 : Constant  Value=zeros(2*Nwheels,1)
  Constant3 : Constant  Value=4
  Gain3 : Gain  Gain=1/sw_tau_2_curr
  Inverse Kinematics 4SW : Subsystem
  Multiport Switch : MultiPortSwitch  DataPortOrder=Zero-based contiguous  Inputs=4
  Own Constrainst Calculator : MATLAB Function  TreatAsAtomicUnit=on
  ROPOD 4SW : Subsystem
  Switch1 : Switch  Criteria=u2 > Threshold
  To File1 : ToFile  Commented=on  Filename=varphi_tau_setp.mat  MatrixName=varphi_tau_setp
  To File2 : ToFile  Commented=on  Filename=varphi_tau_setp_distr  MatrixName=varphi_tau_setp_distr
  Torque distribution : Subsystem
  pivot damping cntr : Subsystem
  wheel flip compensation : Subsystem
  wheel vel cntr : Subsystem
  SW1_cmd : Outport
  SW2_cmd : Outport  Port=2
  SW3_cmd : Outport  Port=3
  SW4_cmd : Outport  Port=4
  enable_robot : Outport  Port=5
  constraints_robot : Outport  Port=6
  wires:
  ROPOD 4SW/4(SW4_cmd) -> SW4_cmd/1
  w_platform_setp/1 -> Torque distribution/1(w_platform_setp)
  ropod_kinmodel_pv/1 -> [ropod_kin_param], Torque distribution/2(ropod_kinmodel_pv)
  ROPOD 4SW/1(SW1_cmd) -> SW1_cmd/1
  ena_w/1 -> [ena_sw], Torque distribution/5(ena_w)
  ROPOD 4SW/3(SW3_cmd) -> SW3_cmd/1
  [sw_conf] -> ROPOD 4SW/1(sw_conf)
  ROPOD 4SW/2(SW2_cmd) -> SW2_cmd/1
  sw_conf/1 -> [sw_conf], Torque distribution/3(sw_conf)
  delta/1 -> [delta], Torque distribution/4(delta)
  [ropod_kin_param] -> wheel flip compensation/2(ropod_kin_param)
  Compare To Constant1/1 -> pivot damping cntr/2(disable)
  ddelta/1 -> pivot damping cntr/4(ddelta)
  [ropod_wheel_cntr_mode] -> Compare To Constant1/1
  platform_ddelta_cntr_param/1 -> pivot damping cntr/1(platform_ddelta_cntr_param)
  [ena_sw] -> pivot damping cntr/5(ena_w)
  Constant/1 -> pivot damping cntr/3(ddelta_ref)
  Torque distribution/1(varphi_tau_setp_out) -> To File2/1, wheel flip compensation/1(varphi_tau_sp_in)
  [sw_conf] -> wheel flip compensation/4(sw_conf)
  [ena_sw] -> Own Constrainst Calculator/3(ena_sw)
  Bus Selector1/1 -> Gain3/1  "<max_current>"
  [sw_conf] -> Bus Selector1/1
  Gain3/1 -> Own Constrainst Calculator/2(tau_max)
  Own Constrainst Calculator/1(enable_local_robot) -> enable_robot/1
  Own Constrainst Calculator/2(constraints_local_robot) -> constraints_robot/1
  [ropod_kin_param] -> Own Constrainst Calculator/1(ropod_kinmodel_param_vec)
  Inverse Kinematics 4SW/1(wheel_vel_sp) -> wheel vel cntr/3(dvarphi_sp)
  [ropod_kin_param] -> Inverse Kinematics 4SW/1(param_in)
  wheel vel cntr/1(varphi_tau_setp_out) -> [varphi_tau_dvarphi_cntr]
  platform_dvarphi_cntr_param/1 -> wheel vel cntr/1(platform_dxdy_cntr_param)
  dqr_sp_dvarphi_cntr/1 -> Inverse Kinematics 4SW/2(dqr_sp)
  dvarphi/1 -> wheel vel cntr/5(dvarphi)
  [ena_sw] -> wheel vel cntr/4(ena_w)
  ropod_cntr_mode/1 -> [ropod_cntr_mode]
  [ropod_cntr_mode] -> ROPOD 4SW/2(ropod_cntr_mode)
  [ropod_wheel_cntr_mode] -> Compare To Constant/1
  Compare To Constant/1 -> wheel vel cntr/2(disable)
  ropod_wheel_cntr_mode/1 -> [ropod_wheel_cntr_mode]
  [delta] -> Inverse Kinematics 4SW/3(delta)
  [ropod_wheel_cntr_mode] -> Compare To Constant2/1
  Constant3/1 -> Switch1/1
  Constant1/1 -> Switch1/3
  Switch1/1 -> wheel flip compensation/3(flip_comp_factor)
  [ropod_wheel_cntr_mode] -> Multiport Switch/1
  Compare To Constant2/1 -> Switch1/2
  pivot damping cntr/1(varphi_tau_setp_out) -> [varphi_tau_ddelta_cntr]
  wheel flip compensation/1(varphi_tau_sp_out) -> Add/1
  Multiport Switch/1 -> Add/2
  Add/1 -> To File1/1, ROPOD 4SW/3(varphi_tau_setp)
  Constant2/1 -> Multiport Switch/2
  [varphi_tau_ddelta_cntr] -> Multiport Switch/3
  [varphi_tau_dvarphi_cntr] -> Multiport Switch/4
  [varphi_tau_ddelta_cntr] -> Multiport Switch/5

== system ROPOD_Control_Control_SIM/Send_configuration_agent ==
  agent_number : Inport
  local_agent_configuration : Inport  Port=2
  Enable : EnablePort
  UDP Send : dspnetwork/UDP Send  remoteURL='255.255.255.255'  remotePort=25002  localURL='0.0.0.0'  localPortSource=Automatically determine  localPort=-1  sampletime=-1  blockPlatform=[]  separateLengthPort=0
      settings: SourceProductName=DSP System Toolbox  SourceProductBaseCode=DS
  Vector Concatenate : Concatenate
  wires:
  agent_number/1 -> Vector Concatenate/1
  local_agent_configuration/1 -> Vector Concatenate/2
  Vector Concatenate/1 -> UDP Send/1

== system ROPOD_Control_Control_SIM/Send_wrench_agents ==
  w_agents_setp : Inport
  Enable : EnablePort
  UDP Send : dspnetwork/UDP Send  remoteURL='255.255.255.255'  remotePort=25001  localURL='0.0.0.0'  localPortSource=Automatically determine  localPort=-1  sampletime=-1  blockPlatform=[]  separateLengthPort=0
      settings: SourceProductName=DSP System Toolbox  SourceProductBaseCode=DS
  wires:
  w_agents_setp/1 -> UDP Send/1

== system ROPOD_Control_Control_SIM/Subsystem ==
  Ropod kinematic parameters : Subsystem
  Smart wheels conf1 : Subsystem
  ropod_kin_param : Outport
  sw_conf : Outport  Port=2
  wires:
  Ropod kinematic parameters/1(ropod_kin_param) -> ropod_kin_param/1
  Smart wheels conf1/1(sw_conf) -> sw_conf/1

== system ROPOD_Control_Control_SIM/to_ROS empty ==
  odom_robot_pose : Inport
  odom_robot_twist : Inport  Port=2
  Terminator1 : Terminator
  Terminator2 : Terminator
  wires:
  odom_robot_pose/1 -> Terminator2/1
  odom_robot_twist/1 -> Terminator1/1

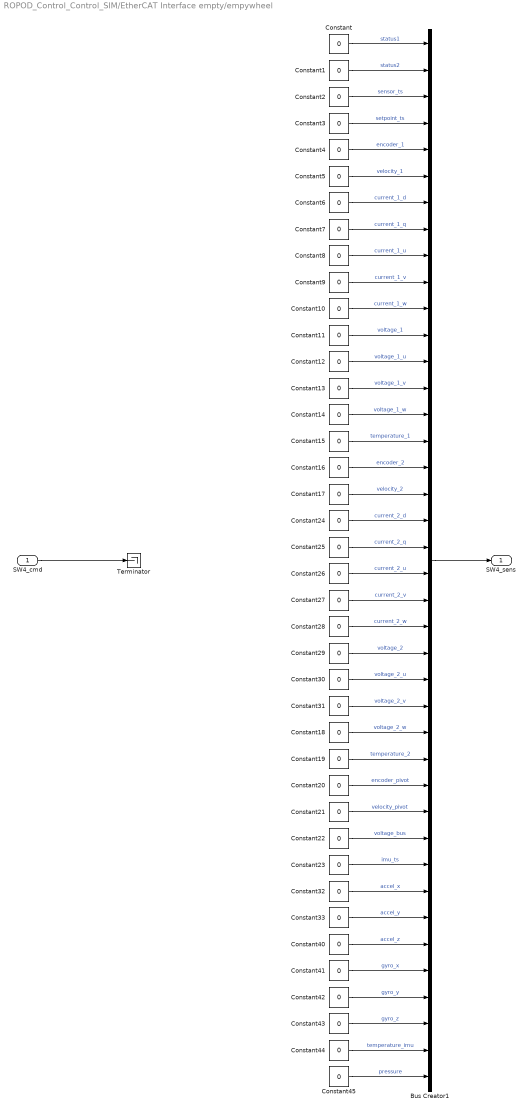
== system ROPOD_Control_Control_SIM/EtherCAT Interface empty/empywheel ==
  SW4_cmd : Inport
  Bus Creator1 : BusCreator  Inputs=40
  Constant{,1..33,40..45} (40 alike) : Constant  Value=0
  Terminator : Terminator
  SW4_sens : Outport
  wires:
  SW4_cmd/1 -> Terminator/1
  Constant23/1 -> Bus Creator1/32  "imu_ts"
  Constant22/1 -> Bus Creator1/31  "voltage_bus"
  Constant7/1 -> Bus Creator1/8  "current_1_q"
  Constant31/1 -> Bus Creator1/26  "voltage_2_v"
  Constant32/1 -> Bus Creator1/33  "accel_x"
  Constant15/1 -> Bus Creator1/16  "temperature_1"
  Constant44/1 -> Bus Creator1/39  "temperature_imu"
  Constant9/1 -> Bus Creator1/10  "current_1_v"
  Constant21/1 -> Bus Creator1/30  "velocity_pivot"
  Constant45/1 -> Bus Creator1/40  "pressure"
  Constant10/1 -> Bus Creator1/11  "current_1_w"
  Constant16/1 -> Bus Creator1/17  "encoder_2"
  Constant3/1 -> Bus Creator1/4  "setpoint_ts"
  Constant28/1 -> Bus Creator1/23  "current_2_w"
  Constant41/1 -> Bus Creator1/36  "gyro_x"
  Constant4/1 -> Bus Creator1/5  "encoder_1"
  Constant6/1 -> Bus Creator1/7  "current_1_d"
  Constant18/1 -> Bus Creator1/27  "voltage_2_w"
  Constant12/1 -> Bus Creator1/13  "voltage_1_u"
  Constant43/1 -> Bus Creator1/38  "gyro_z"
  Constant25/1 -> Bus Creator1/20  "current_2_q"
  Constant42/1 -> Bus Creator1/37  "gyro_y"
  Constant19/1 -> Bus Creator1/28  "temperature_2"
  Constant8/1 -> Bus Creator1/9  "current_1_u"
  Constant14/1 -> Bus Creator1/15  "voltage_1_w"
  Constant29/1 -> Bus Creator1/24  "voltage_2"
  Constant30/1 -> Bus Creator1/25  "voltage_2_u"
  Constant27/1 -> Bus Creator1/22  "current_2_v"
  Constant/1 -> Bus Creator1/1  "status1"
  Constant1/1 -> Bus Creator1/2  "status2"
  Constant40/1 -> Bus Creator1/35  "accel_z"
  Constant11/1 -> Bus Creator1/12  "voltage_1"
  Constant5/1 -> Bus Creator1/6  "velocity_1"
  Constant13/1 -> Bus Creator1/14  "voltage_1_v"
  Constant24/1 -> Bus Creator1/19  "current_2_d"
  Constant17/1 -> Bus Creator1/18  "velocity_2"
  Constant20/1 -> Bus Creator1/29  "encoder_pivot"
  Constant33/1 -> Bus Creator1/34  "accel_y"
  Constant2/1 -> Bus Creator1/3  "sensor_ts"
  Constant26/1 -> Bus Creator1/21  "current_2_u"
  Bus Creator1/1 -> SW4_sens/1

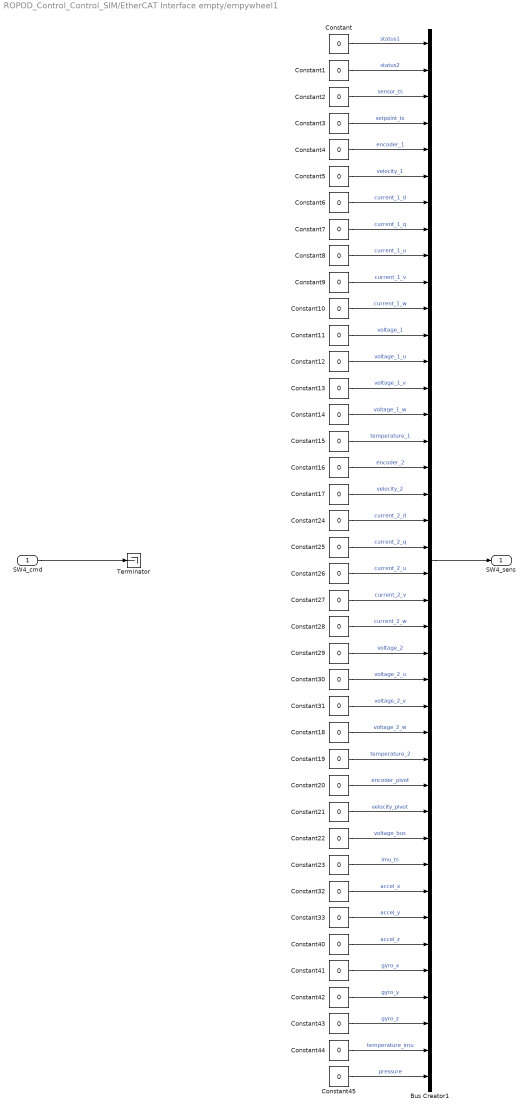
== system ROPOD_Control_Control_SIM/EtherCAT Interface empty/empywheel1 ==
  SW4_cmd : Inport
  Bus Creator1 : BusCreator  Inputs=40
  Constant{,1..33,40..45} (40 alike) : Constant  Value=0
  Terminator : Terminator
  SW4_sens : Outport
  wires:
  Bus Creator1/1 -> SW4_sens/1
  Constant26/1 -> Bus Creator1/21  "current_2_u"
  Constant2/1 -> Bus Creator1/3  "sensor_ts"
  Constant33/1 -> Bus Creator1/34  "accel_y"
  Constant20/1 -> Bus Creator1/29  "encoder_pivot"
  Constant17/1 -> Bus Creator1/18  "velocity_2"
  Constant24/1 -> Bus Creator1/19  "current_2_d"
  Constant13/1 -> Bus Creator1/14  "voltage_1_v"
  Constant5/1 -> Bus Creator1/6  "velocity_1"
  Constant11/1 -> Bus Creator1/12  "voltage_1"
  Constant40/1 -> Bus Creator1/35  "accel_z"
  Constant1/1 -> Bus Creator1/2  "status2"
  Constant/1 -> Bus Creator1/1  "status1"
  Constant27/1 -> Bus Creator1/22  "current_2_v"
  Constant30/1 -> Bus Creator1/25  "voltage_2_u"
  Constant29/1 -> Bus Creator1/24  "voltage_2"
  Constant14/1 -> Bus Creator1/15  "voltage_1_w"
  Constant8/1 -> Bus Creator1/9  "current_1_u"
  Constant19/1 -> Bus Creator1/28  "temperature_2"
  Constant42/1 -> Bus Creator1/37  "gyro_y"
  Constant25/1 -> Bus Creator1/20  "current_2_q"
  Constant43/1 -> Bus Creator1/38  "gyro_z"
  Constant12/1 -> Bus Creator1/13  "voltage_1_u"
  Constant18/1 -> Bus Creator1/27  "voltage_2_w"
  Constant6/1 -> Bus Creator1/7  "current_1_d"
  Constant4/1 -> Bus Creator1/5  "encoder_1"
  Constant41/1 -> Bus Creator1/36  "gyro_x"
  Constant28/1 -> Bus Creator1/23  "current_2_w"
  Constant3/1 -> Bus Creator1/4  "setpoint_ts"
  Constant16/1 -> Bus Creator1/17  "encoder_2"
  Constant10/1 -> Bus Creator1/11  "current_1_w"
  Constant45/1 -> Bus Creator1/40  "pressure"
  Constant21/1 -> Bus Creator1/30  "velocity_pivot"
  Constant9/1 -> Bus Creator1/10  "current_1_v"
  Constant44/1 -> Bus Creator1/39  "temperature_imu"
  Constant15/1 -> Bus Creator1/16  "temperature_1"
  Constant32/1 -> Bus Creator1/33  "accel_x"
  Constant31/1 -> Bus Creator1/26  "voltage_2_v"
  Constant7/1 -> Bus Creator1/8  "current_1_q"
  Constant22/1 -> Bus Creator1/31  "voltage_bus"
  Constant23/1 -> Bus Creator1/32  "imu_ts"
  SW4_cmd/1 -> Terminator/1

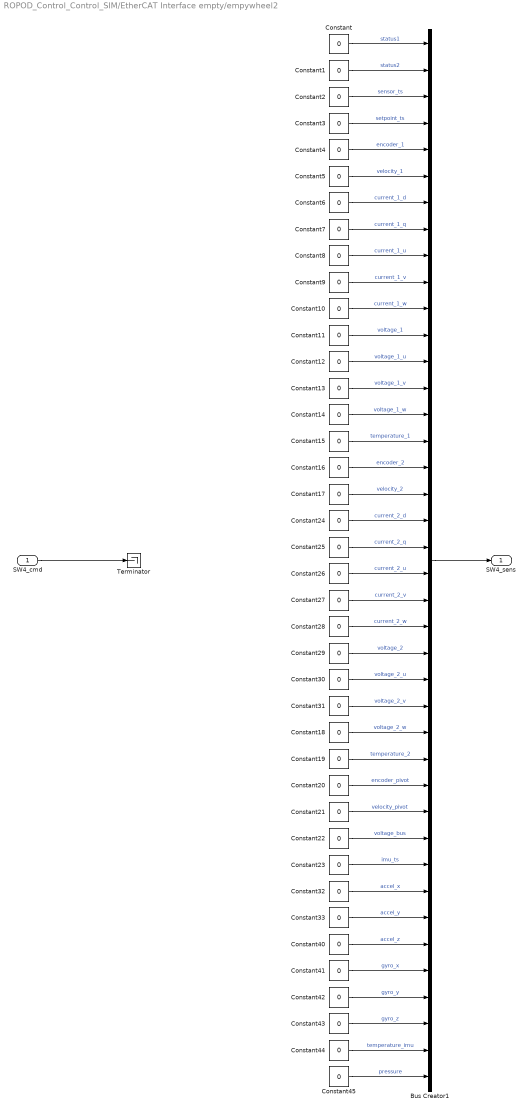
== system ROPOD_Control_Control_SIM/EtherCAT Interface empty/empywheel2 ==
  SW4_cmd : Inport
  Bus Creator1 : BusCreator  Inputs=40
  Constant{,1..33,40..45} (40 alike) : Constant  Value=0
  Terminator : Terminator
  SW4_sens : Outport
  wires:
  SW4_cmd/1 -> Terminator/1
  Constant23/1 -> Bus Creator1/32  "imu_ts"
  Constant22/1 -> Bus Creator1/31  "voltage_bus"
  Constant7/1 -> Bus Creator1/8  "current_1_q"
  Constant31/1 -> Bus Creator1/26  "voltage_2_v"
  Constant32/1 -> Bus Creator1/33  "accel_x"
  Constant15/1 -> Bus Creator1/16  "temperature_1"
  Constant44/1 -> Bus Creator1/39  "temperature_imu"
  Constant9/1 -> Bus Creator1/10  "current_1_v"
  Constant21/1 -> Bus Creator1/30  "velocity_pivot"
  Constant45/1 -> Bus Creator1/40  "pressure"
  Constant10/1 -> Bus Creator1/11  "current_1_w"
  Constant16/1 -> Bus Creator1/17  "encoder_2"
  Constant3/1 -> Bus Creator1/4  "setpoint_ts"
  Constant28/1 -> Bus Creator1/23  "current_2_w"
  Constant41/1 -> Bus Creator1/36  "gyro_x"
  Constant4/1 -> Bus Creator1/5  "encoder_1"
  Constant6/1 -> Bus Creator1/7  "current_1_d"
  Constant18/1 -> Bus Creator1/27  "voltage_2_w"
  Constant12/1 -> Bus Creator1/13  "voltage_1_u"
  Constant43/1 -> Bus Creator1/38  "gyro_z"
  Constant25/1 -> Bus Creator1/20  "current_2_q"
  Constant42/1 -> Bus Creator1/37  "gyro_y"
  Constant19/1 -> Bus Creator1/28  "temperature_2"
  Constant8/1 -> Bus Creator1/9  "current_1_u"
  Constant14/1 -> Bus Creator1/15  "voltage_1_w"
  Constant29/1 -> Bus Creator1/24  "voltage_2"
  Constant30/1 -> Bus Creator1/25  "voltage_2_u"
  Constant27/1 -> Bus Creator1/22  "current_2_v"
  Constant/1 -> Bus Creator1/1  "status1"
  Constant1/1 -> Bus Creator1/2  "status2"
  Constant40/1 -> Bus Creator1/35  "accel_z"
  Constant11/1 -> Bus Creator1/12  "voltage_1"
  Constant5/1 -> Bus Creator1/6  "velocity_1"
  Constant13/1 -> Bus Creator1/14  "voltage_1_v"
  Constant24/1 -> Bus Creator1/19  "current_2_d"
  Constant17/1 -> Bus Creator1/18  "velocity_2"
  Constant20/1 -> Bus Creator1/29  "encoder_pivot"
  Constant33/1 -> Bus Creator1/34  "accel_y"
  Constant2/1 -> Bus Creator1/3  "sensor_ts"
  Constant26/1 -> Bus Creator1/21  "current_2_u"
  Bus Creator1/1 -> SW4_sens/1

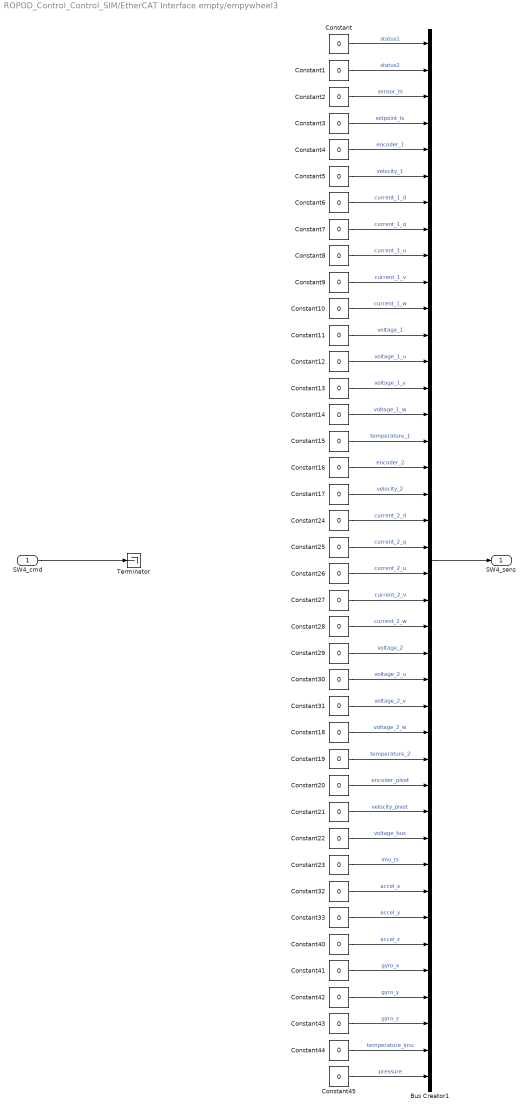
== system ROPOD_Control_Control_SIM/EtherCAT Interface empty/empywheel3 ==
  SW4_cmd : Inport
  Bus Creator1 : BusCreator  Inputs=40
  Constant{,1..33,40..45} (40 alike) : Constant  Value=0
  Terminator : Terminator
  SW4_sens : Outport
  wires:
  Bus Creator1/1 -> SW4_sens/1
  Constant26/1 -> Bus Creator1/21  "current_2_u"
  Constant2/1 -> Bus Creator1/3  "sensor_ts"
  Constant33/1 -> Bus Creator1/34  "accel_y"
  Constant20/1 -> Bus Creator1/29  "encoder_pivot"
  Constant17/1 -> Bus Creator1/18  "velocity_2"
  Constant24/1 -> Bus Creator1/19  "current_2_d"
  Constant13/1 -> Bus Creator1/14  "voltage_1_v"
  Constant5/1 -> Bus Creator1/6  "velocity_1"
  Constant11/1 -> Bus Creator1/12  "voltage_1"
  Constant40/1 -> Bus Creator1/35  "accel_z"
  Constant1/1 -> Bus Creator1/2  "status2"
  Constant/1 -> Bus Creator1/1  "status1"
  Constant27/1 -> Bus Creator1/22  "current_2_v"
  Constant30/1 -> Bus Creator1/25  "voltage_2_u"
  Constant29/1 -> Bus Creator1/24  "voltage_2"
  Constant14/1 -> Bus Creator1/15  "voltage_1_w"
  Constant8/1 -> Bus Creator1/9  "current_1_u"
  Constant19/1 -> Bus Creator1/28  "temperature_2"
  Constant42/1 -> Bus Creator1/37  "gyro_y"
  Constant25/1 -> Bus Creator1/20  "current_2_q"
  Constant43/1 -> Bus Creator1/38  "gyro_z"
  Constant12/1 -> Bus Creator1/13  "voltage_1_u"
  Constant18/1 -> Bus Creator1/27  "voltage_2_w"
  Constant6/1 -> Bus Creator1/7  "current_1_d"
  Constant4/1 -> Bus Creator1/5  "encoder_1"
  Constant41/1 -> Bus Creator1/36  "gyro_x"
  Constant28/1 -> Bus Creator1/23  "current_2_w"
  Constant3/1 -> Bus Creator1/4  "setpoint_ts"
  Constant16/1 -> Bus Creator1/17  "encoder_2"
  Constant10/1 -> Bus Creator1/11  "current_1_w"
  Constant45/1 -> Bus Creator1/40  "pressure"
  Constant21/1 -> Bus Creator1/30  "velocity_pivot"
  Constant9/1 -> Bus Creator1/10  "current_1_v"
  Constant44/1 -> Bus Creator1/39  "temperature_imu"
  Constant15/1 -> Bus Creator1/16  "temperature_1"
  Constant32/1 -> Bus Creator1/33  "accel_x"
  Constant31/1 -> Bus Creator1/26  "voltage_2_v"
  Constant7/1 -> Bus Creator1/8  "current_1_q"
  Constant22/1 -> Bus Creator1/31  "voltage_bus"
  Constant23/1 -> Bus Creator1/32  "imu_ts"
  SW4_cmd/1 -> Terminator/1

== system ROPOD_Control_Control_SIM/Flock_Control/Flock Velocity controller ==
  note: Mass Feedforward
  disable : Inport
  flock_dxdy_cntr_param : Inport  Port=2
  flock_dtheta_cntr_param : Inport  Port=3
  dq_flock_sp : Inport  Port=4
  dq_flock_loc : Inport  Port=5
  Compare To Constant : simulink/Logic and Bit Operations/Compare To Constant  relop===  const=0  OutDataTypeStr=boolean
  Compare To Constant1 : simulink/Logic and Bit Operations/Compare To Constant  relop===  const=0  OutDataTypeStr=boolean
  Demux : Demux  Outputs=3
  Demux1 : Demux  Outputs=3
  G_I_LL_LPF Controller_flock_Theta : Subsystem
  G_I_LL_LPF Controller_flock_X : Subsystem
  G_I_LL_LPF Controller_flock_Y : Subsystem
  Gain : Gain  Gain=flock_FFxy_friction
  Gain1 : Gain  Gain=flock_FFxy_friction
  Gain2 : Gain  Gain=flock_FFtheta_friction
  Mux : Mux  Inputs=3
  Mux1 : Mux  Inputs=3
  Product : Product
  Product1 : Product
  Sign : Signum
  Sum : Sum  Inputs=|+-
  Sum1 : Sum  Inputs=++|
  w_flock_setp : Outport
  wires:
  G_I_LL_LPF Controller_flock_Theta/1(Out) -> Mux/3
  Demux/1 -> G_I_LL_LPF Controller_flock_X/2(In)
  Demux/2 -> G_I_LL_LPF Controller_flock_Y/2(In)
  G_I_LL_LPF Controller_flock_Y/1(Out) -> Mux/2
  G_I_LL_LPF Controller_flock_X/1(Out) -> Mux/1
  Demux/3 -> G_I_LL_LPF Controller_flock_Theta/2(In)
  dq_flock_sp/1 -> Sign/1, Sum/1
  dq_flock_loc/1 -> Sum/2
  [param_dxdy_cntr] -> G_I_LL_LPF Controller_flock_X/1(param)
  [param_dxdy_cntr] -> G_I_LL_LPF Controller_flock_Y/1(param)
  [param_dtheta_cntr] -> G_I_LL_LPF Controller_flock_Theta/1(param)
  disable/1 -> [disable]
  [disable] -> G_I_LL_LPF Controller_flock_X/3(reset_integrator)
  [disable] -> G_I_LL_LPF Controller_flock_Y/3(reset_integrator)
  flock_dxdy_cntr_param/1 -> [param_dxdy_cntr]
  flock_dtheta_cntr_param/1 -> [param_dtheta_cntr]
  [disable] -> G_I_LL_LPF Controller_flock_Theta/3(reset_integrator)
  Sign/1 -> Demux1/1
  Demux1/1 -> Gain/1
  Gain/1 -> Mux1/1
  Demux1/2 -> Gain1/1
  Gain1/1 -> Mux1/2
  Demux1/3 -> Gain2/1
  Gain2/1 -> Mux1/3
  Mux1/1 -> Sum1/1
  Mux/1 -> Sum1/2
  Sum/1 -> Product/1
  Product/1 -> Demux/1
  Compare To Constant/1 -> Product/2
  [disable] -> Compare To Constant/1
  [disable] -> Compare To Constant1/1
  Sum1/1 -> Product1/1
  Compare To Constant1/1 -> Product1/2
  Product1/1 -> w_flock_setp/1
